simulink model "matrices_mat_fct_simulink"  (R2017a)
settings: Solver=VariableStepAuto  StartTime=0.0  StopTime=10.0  RelTol=1e-3
settings Model: Creator=clizo  LastModifiedBy=clizo

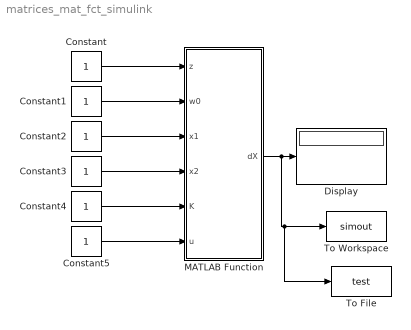
== system matrices_mat_fct_simulink ==
  Constant{,1..5} (6 alike) : Constant
  Display : Display
  MATLAB Function : MATLAB Function  TreatAsAtomicUnit=on
  To File : ToFile  Filename=test  SaveFormat=Timeseries
  To Workspace : ToWorkspace  VariableName=simout  SaveFormat=Timeseries  SampleTime=-1
  wires:
  Constant/1 -> MATLAB Function/1(z)
  Constant5/1 -> MATLAB Function/6(u)
  Constant4/1 -> MATLAB Function/5(K)
  Constant3/1 -> MATLAB Function/4(x2)
  Constant2/1 -> MATLAB Function/3(x1)
  Constant1/1 -> MATLAB Function/2(w0)
  MATLAB Function/1(dX) -> To File/1, To Workspace/1, Display/1

== matlab function matrices_mat_fct_simulink/MATLAB Function ==
  data: z input; w0 input; x1 input; x2 input; K input; u input; dX output
function dX = fcn(z,w0,x1,x2,K,u)

A = [-2*z*w0 -w0^2; 1 0];
X = [x1; x2];
B = [K*w0^2; 0];

dX = A*X+B*u;
